simulink model "LQ_Kalman_LQG"  (R2022b)
settings: Solver=VariableStepAuto  StartTime=0.0  StopTime=15.0  RelTol=1e-3
undefined symbols (not defined in the file or in its folder): A, A_osservatore, B, B_osservatore, C, C_osservatore, D_osservatore, D_process, Klqi, Klqp
libraries: simulink x6
settings Model: Creator=emanuela  LastModifiedBy=emanuela
settings DataIOCC: SaveOutput=off  SignalLogging=off  DSMLogging=off  SaveTime=off  ReturnWorkspaceOutputs=off

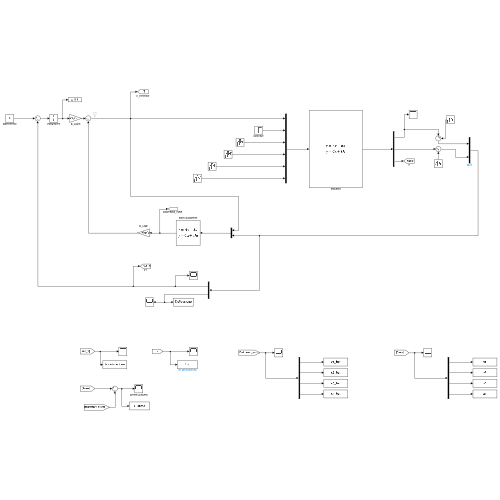
[thumbnail: Simulink's stored preview of the top-level diagram]
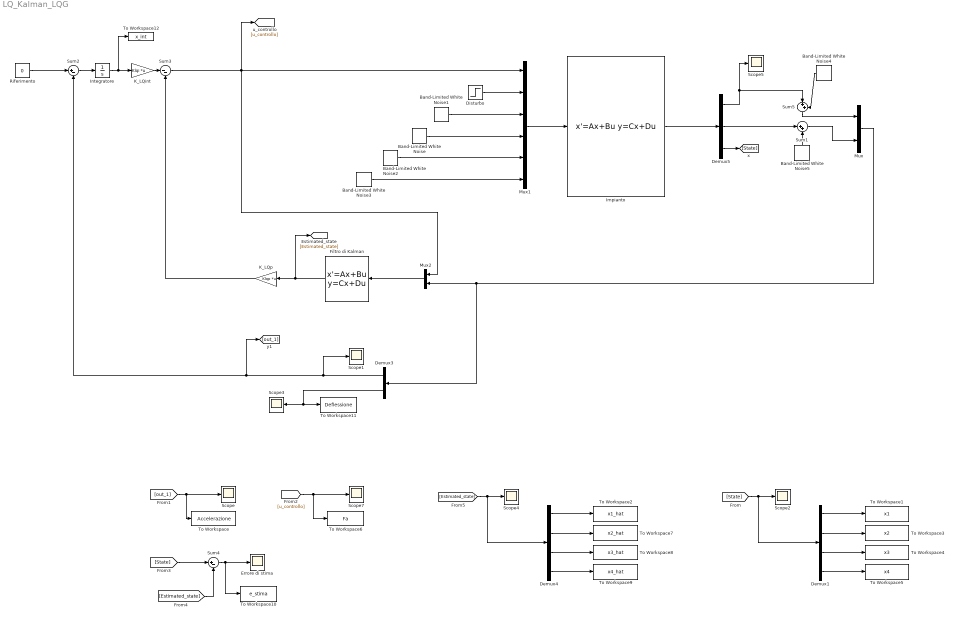
== system LQ_Kalman_LQG ==
  Band-Limited White Noise : simulink/Sources/Band-Limited White Noise  Cov=Pw2  Ts=0.01  seed=[2345]
  Band-Limited White Noise1 : simulink/Sources/Band-Limited White Noise  Cov=Pw1  Ts=0.01  seed=[2345]
  Band-Limited White Noise2 : simulink/Sources/Band-Limited White Noise  Cov=Pw3  Ts=0.01  seed=[3456]
  Band-Limited White Noise3 : simulink/Sources/Band-Limited White Noise  Cov=Pw4  Ts=0.01  seed=[4567]
  Band-Limited White Noise4 : simulink/Sources/Band-Limited White Noise  Cov=Pv_acc  Ts=0.01  seed=[5678]
  Band-Limited White Noise5 : simulink/Sources/Band-Limited White Noise  Cov=Pv_acc  Ts=0.01  seed=[5678]
  Demux1 : Demux
  Demux3 : Demux  Outputs=2
  Demux4 : Demux
  Demux5 : Demux  Outputs=3
  Disturbo : Step  After=0.05  SampleTime=0
  Errore di stima : Scope
  Filtro di Kalman : StateSpace  A=A_osservatore  B=B_osservatore  C=C_osservatore  D=D_osservatore  InitialCondition=0 * ones(4,1);
  Impianto : StateSpace  A=A  B=[B, eye(4)]  C=[C; eye(4)]  D=[D_process ; zeros(4,6)]  InitialCondition=0
  Integratore : Integrator
  K_LQint : Gain  Gain=Klqi  Multiplication=Matrix(K*u)
  K_LQp : Gain  Gain=Klqp  Multiplication=Matrix(K*u)
  Mux : Mux  Inputs=2
  Mux1 : Mux  Inputs=6
  Mux2 : Mux  Inputs=2
  Riferimento : Constant  Value=0
  Scope{,1..5,7} (7 alike) : Scope
  Sum1 : Sum  Inputs=|++
  Sum2 : Sum  Inputs=|+-
  Sum3 : Sum  Inputs=|--
  Sum4 : Sum  Inputs=|+-
  Sum5 : Sum  Inputs=|++
  To Workspace : ToWorkspace  VariableName=Accelerazione  SaveFormat=Timeseries  SampleTime=-1
  To Workspace1 : ToWorkspace  VariableName=x1  SaveFormat=Timeseries  SampleTime=-1
  To Workspace10 : ToWorkspace  VariableName=e_stima  SaveFormat=Timeseries  SampleTime=-1
  To Workspace11 : ToWorkspace  VariableName=Deflessione  SaveFormat=Timeseries  SampleTime=-1
  To Workspace12 : ToWorkspace  VariableName=x_int  SaveFormat=Timeseries  SampleTime=-1
  To Workspace2 : ToWorkspace  VariableName=x1_hat  SaveFormat=Timeseries  SampleTime=-1
  To Workspace3 : ToWorkspace  VariableName=x2  SaveFormat=Timeseries  SampleTime=-1
  To Workspace4 : ToWorkspace  VariableName=x3  SaveFormat=Timeseries  SampleTime=-1
  To Workspace5 : ToWorkspace  VariableName=x4  SaveFormat=Timeseries  SampleTime=-1
  To Workspace6 : ToWorkspace  VariableName=Fa  SaveFormat=Timeseries  SampleTime=-1
  To Workspace7 : ToWorkspace  VariableName=x2_hat  SaveFormat=Timeseries  SampleTime=-1
  To Workspace8 : ToWorkspace  VariableName=x3_hat  SaveFormat=Timeseries  SampleTime=-1
  To Workspace9 : ToWorkspace  VariableName=x4_hat  SaveFormat=Timeseries  SampleTime=-1
  wires:
  K_LQint/1 -> Sum3/1
  [out_1] -> To Workspace/1, Scope/1
  [Estimated_state] -> Sum4/2
  Integratore/1 -> To Workspace12/1, K_LQint/1
  Demux3/2 -> Scope3/1, To Workspace11/1
  Riferimento/1 -> Sum2/1
  Mux2/1 -> Filtro di Kalman/1
  Mux1/1 -> Impianto/1
  Demux3/1 -> Scope1/1, [out_1], Sum2/2
  Sum3/1 -> Mux2/1, [u_controllo], Mux1/1
  Disturbo/1 -> Mux1/2
  [Estimated_state] -> Demux4/1, Scope4/1
  [State] -> Sum4/1
  Sum4/1 -> To Workspace10/1, Errore di stima/1
  K_LQp/1 -> Sum3/2
  Demux4/3 -> To Workspace8/1
  Demux4/1 -> To Workspace2/1
  [u_controllo] -> Scope7/1, To Workspace6/1
  Sum2/1 -> Integratore/1
  Filtro di Kalman/1 -> K_LQp/1, [Estimated_state]
  Demux4/4 -> To Workspace9/1
  Demux4/2 -> To Workspace7/1
  Band-Limited White Noise1/1 -> Mux1/3
  Band-Limited White Noise/1 -> Mux1/4
  Band-Limited White Noise2/1 -> Mux1/5
  Band-Limited White Noise3/1 -> Mux1/6
  Band-Limited White Noise5/1 -> Sum1/2
  Demux5/2 -> Sum1/1
  Mux/1 -> Demux3/1, Mux2/2
  Impianto/1 -> Demux5/1
  Demux5/1 -> Scope5/1, Sum5/1
  Band-Limited White Noise4/1 -> Sum5/2
  Sum5/1 -> Mux/1
  Sum1/1 -> Mux/2
  Demux5/3 -> [State]
  Demux1/3 -> To Workspace4/1
  Demux1/2 -> To Workspace3/1
  [State] -> Demux1/1, Scope2/1
  Demux1/4 -> To Workspace5/1
  Demux1/1 -> To Workspace1/1
